simulink model "kpkdki"  (R2014a)
settings: Solver=ode3  StartTime=0.0  StopTime=10.0  FixedStep=.01  RelTol=1e-3
values from neighbouring files (symbols this model uses):
  a = 21    [blackbox_step_graph.m]    (also in working.mat)
settings Model: Creator=gabriellemerritt  LastModifiedBy=gabriellemerritt

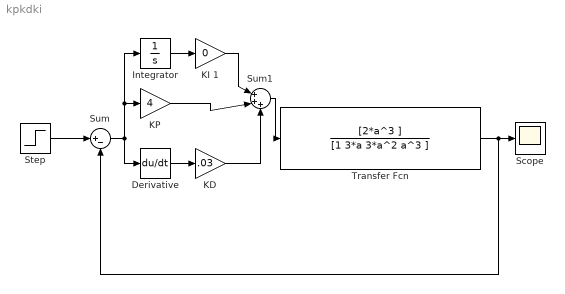
== system kpkdki ==
  Derivative : Derivative
  Integrator : Integrator
  "KD " : Gain  Gain=.03
  KI 1 : Gain  Gain=0
  KP : Gain  Gain=4
  Scope : Scope
      settings: TickLabels=on  TimeRange=3  YMin=0  YMax=1.8  SaveName=ScopeData2
  Step : Step  SampleTime=0
  Sum : Sum  Inputs=|+-
  Sum1 : Sum  Inputs=|+++
  Transfer Fcn : TransferFcn  Numerator=[2*a^3 ]  Denominator=[1 3*a 3*a^2 a^3 ]
  wires:
  Transfer Fcn/1 -> Scope/1, Sum/2
  Step/1 -> Sum/1
  Sum/1 -> Derivative/1, Integrator/1, KP/1
  Derivative/1 -> "KD "/1
  Sum1/1 -> Transfer Fcn/1
  Integrator/1 -> KI 1/1
  KI 1/1 -> Sum1/1
  KP/1 -> Sum1/2
  "KD "/1 -> Sum1/3
